simulink model "minta2007_02_05"  (R2013a)
settings: Solver=ode45  StartTime=0.0  StopTime=50  RelTol=1e-3
undefined symbols (not defined in the file or in its folder): Ad, Bd, Cd, Dd, F, G, H, K, Nu, Nx, Ts
settings Model: Creator=rudi  LastModifiedBy=rudi

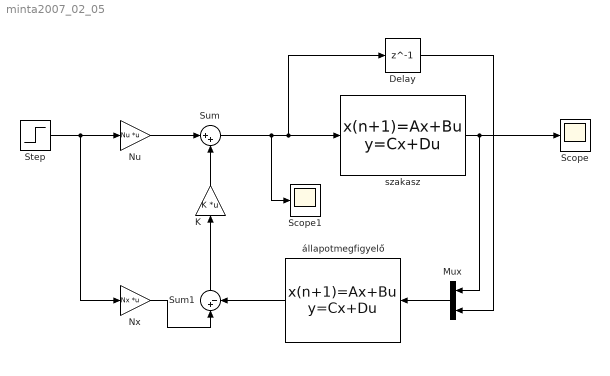
== system minta2007_02_05 ==
  Delay : Delay  DelayLength=1  SampleTime=Ts
  K : Gain  Gain=K  Multiplication=Matrix(K*u)
  Mux : Mux  Inputs=2
  Nu : Gain  Gain=Nu  Multiplication=Matrix(K*u)
  Nx : Gain  Gain=Nx  Multiplication=Matrix(K*u)
  Scope : Scope
  Scope1 : Scope
  Step : Step  SampleTime=0
  Sum : Sum  Inputs=|++
  Sum1 : Sum  Inputs=|+-
  szakasz : DiscreteStateSpace  A=Ad  B=Bd  C=Cd  D=Dd
  állapotmegfigyelő : DiscreteStateSpace  A=F  B=[G, H]  C=eye(2)  D=[0, 0; 0, 0]
  wires:
  állapotmegfigyelő/1 -> Sum1/2
  Nx/1 -> Sum1/1
  Nu/1 -> Sum/1
  K/1 -> Sum/2
  Sum1/1 -> K/1
  Step/1 -> Nx/1, Nu/1
  szakasz/1 -> Scope/1, Mux/1
  Mux/1 -> állapotmegfigyelő/1
  Sum/1 -> Scope1/1, Delay/1, szakasz/1
  Delay/1 -> Mux/2
